simulink model "BasicRobot_RightWheelTest"  (R2023b)
settings: Solver=VariableStepAuto  StartTime=0.0  StopTime=10.0  RelTol=1e-3
values from neighbouring files (symbols this model uses):
  m = 2.5    [BasicRobot_Parameters.m]
settings Model: Creator=BeanieBabyJ  LastModifiedBy=BeanieBabyJ

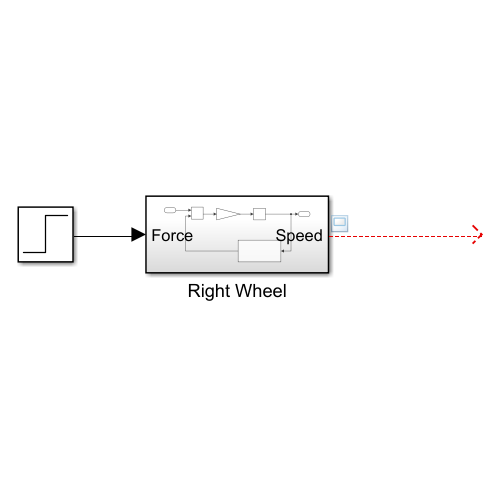
[thumbnail: Simulink's stored preview of the top-level diagram]
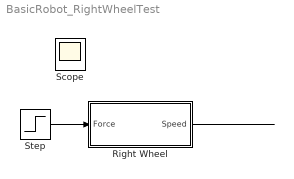
== system BasicRobot_RightWheelTest ==
  Right Wheel : Subsystem
  Step : Step  SampleTime=0
  Scope : Scope
  wires:
  Step/1 -> Right Wheel/1(Force)
  Right Wheel/1(Speed) -> ?

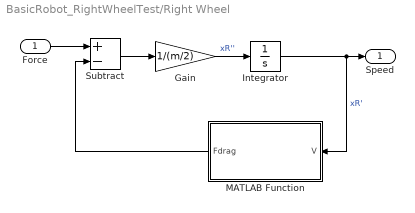
== system BasicRobot_RightWheelTest/Right Wheel ==
  Force : Inport
  Gain : Gain  Gain=1/(m/2)
  Integrator : Integrator
  MATLAB Function : MATLAB Function  TreatAsAtomicUnit=on
  Subtract : Sum  Inputs=+-
  Speed : Outport
  wires:
  Integrator/1 -> MATLAB Function/1(V), Speed/1  "xR'"
  Gain/1 -> Integrator/1  "xR''"
  Force/1 -> Subtract/1
  MATLAB Function/1(Fdrag) -> Subtract/2
  Subtract/1 -> Gain/1

== matlab function BasicRobot_RightWheelTest/Right Wheel/MATLAB Function ==
  data: Fdrag output; V input; k_drag parameter
function Fdrag=get_fdrag(V, k_drag)

Fdrag=k_drag*V*abs(V);
